simulink model "untitled2"  (Simulink 7.6)
settings: Solver=ode4  StartTime=0.0  StopTime=inf  FixedStep=0.2  RelTol=1e-3
undefined symbols (not defined in the file or in its folder): bit, Standard
libraries: xpclib x9, simulink x2
settings Model: xpc_rtwmakecfg_data=_xpccanac2pci_  Creator=Administrator  LastModifiedBy=Administrator  SimulationMode=external  BufferReuse=off
settings OptimizationCC: BlockReduction=off  OptimizeBlockIOStorage=off  BufferReuse=off  ExpressionFolding=off  LocalBlockOutputs=off
settings HardwareCC: ProdIntDivRoundTo=Zero  ProdEndianess=LittleEndian  ProdHWDeviceType=Generic->32-bit x86 compatible
settings RTWCC: SystemTargetFile=xpctarget.tlc  TemplateMakefile=xpc_default_tmf  Description=xPC Target  ProcessScript=xpctarget_make_rtw_hook  RTWCompilerOptimization=On
settings xpcTargetCC: TargetFcnLib=ansi_tfl_table_tmw.mat  TargetFunctionLibrary=XPC_BLAS  ERTCodeCoverageTool=None  ParMdlRefBuildCompliant=on  CombineSignalStateStructs=off  PortableWordSizes=off  xPCLoadParamSetFile=off  xPCConcurrentTasks=off  xPCEnableSFAnimation=off

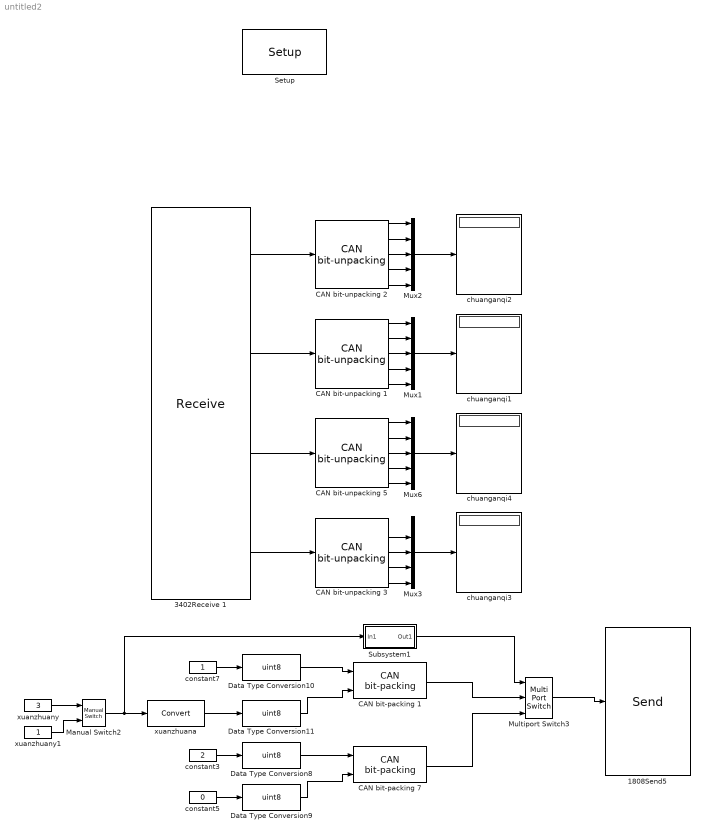
== system untitled2 ==
  1808Send5 : xpclib/CAN/Softing/CAN-AC2-PCI SJA 1000/Send   board=1  canPort=CAN 2  range=Standard (11-bit)  ids=1  sizes=[8]  output=off  ts=-1  ididx=[0]
  3402Receive 1 : xpclib/CAN/Softing/CAN-AC2-PCI SJA 1000/Receive   board=1  canPort=CAN 2  range=Standard (11-bit)  ids=[1 2 3 4]  lengths=8  output=Data  inten=off  ts=-1  ididx=[0,1,2,3]
  CAN bit-packing 1 : xpclib/CAN/Utilities/CAN bit-packing   bitpatterns={ [0:7] [8:15] }
  CAN bit-packing 7 : xpclib/CAN/Utilities/CAN bit-packing   bitpatterns={ [0:7] [8:15] }
  CAN bit-unpacking {1..3,5} (4 alike) : xpclib/CAN/Utilities/CAN bit-unpacking   bitpatterns={ [0:7],[8:15],[16:23],[24:31],[32:39]}  dtypes={ 'uint8','uint8','uint8','uint8','uint8' }
  Data Type Conversion{8..11} (4 alike) : DataTypeConversion  OutDataTypeStr=uint8
  Manual Switch2 : simulink/Signal Routing/Manual Switch  SystemSampleTime=-1  sw=1  action=0  varsize=off
  Multiport Switch3 : MultiPortSwitch  DataPortOrder=Zero-based contiguous  Inputs=2  zeroidx=on
  Mux{1..3,6} (4 alike) : Mux  Inputs=5
  "Setup " : xpclib/CAN/Softing/CAN-AC2-PCI SJA 1000/Setup   board=1  can1bus=Highspeed (ISO 11898)  can1Baudrate=500 kBaud  can1UserBR=[1,1,4,3]  can2bus=Highspeed (ISO 11898)  can2Baudrate=500 kBaud  can2UserBR=[1,1,4,3]  init=[]  term=[]  bus_off_out=off  bus_off_rec=Off  ioBaseAddress=-1
  Subsystem1 : Subsystem
  chuanganqi{1..4} (4 alike) : Display
  constant3 : Constant  Value=2
  constant5 : Constant  Value=0
  constant7 : Constant
  xuanzhuana : DataTypeConversion
  xuanzhuany : Constant  Value=3
  xuanzhuany1 : Constant
  wires:
  constant7/1 -> Data Type Conversion10/1
  Data Type Conversion10/1 -> CAN bit-packing 1/1
  Data Type Conversion11/1 -> CAN bit-packing 1/2
  constant3/1 -> Data Type Conversion8/1
  Data Type Conversion8/1 -> CAN bit-packing 7/1
  Data Type Conversion9/1 -> CAN bit-packing 7/2
  constant5/1 -> Data Type Conversion9/1
  xuanzhuana/1 -> Data Type Conversion11/1
  Multiport Switch3/1 -> 1808Send5/1
  CAN bit-packing 1/1 -> Multiport Switch3/2
  Subsystem1/1(Out1) -> Multiport Switch3/1
  CAN bit-packing 7/1 -> Multiport Switch3/3
  Manual Switch2/1 -> xuanzhuana/1, Subsystem1/1(In1)
  xuanzhuany/1 -> Manual Switch2/1
  xuanzhuany1/1 -> Manual Switch2/2
  CAN bit-unpacking 5/5 -> Mux6/5
  3402Receive 1/3 -> CAN bit-unpacking 5/1
  CAN bit-unpacking 5/1 -> Mux6/1
  CAN bit-unpacking 5/2 -> Mux6/2
  CAN bit-unpacking 5/3 -> Mux6/3
  CAN bit-unpacking 5/4 -> Mux6/4
  Mux6/1 -> chuanganqi4/1
  CAN bit-unpacking 1/5 -> Mux1/5
  CAN bit-unpacking 1/1 -> Mux1/1
  CAN bit-unpacking 1/2 -> Mux1/2
  CAN bit-unpacking 1/3 -> Mux1/3
  CAN bit-unpacking 1/4 -> Mux1/4
  Mux1/1 -> chuanganqi1/1
  3402Receive 1/2 -> CAN bit-unpacking 1/1
  CAN bit-unpacking 2/5 -> Mux2/5
  CAN bit-unpacking 2/1 -> Mux2/1
  CAN bit-unpacking 2/2 -> Mux2/2
  CAN bit-unpacking 2/3 -> Mux2/3
  CAN bit-unpacking 2/4 -> Mux2/4
  Mux2/1 -> chuanganqi2/1
  3402Receive 1/1 -> CAN bit-unpacking 2/1
  CAN bit-unpacking 3/5 -> Mux3/5
  CAN bit-unpacking 3/2 -> Mux3/2
  CAN bit-unpacking 3/3 -> Mux3/3
  CAN bit-unpacking 3/4 -> Mux3/4
  Mux3/1 -> chuanganqi3/1
  3402Receive 1/4 -> CAN bit-unpacking 3/1

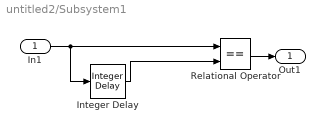
== system untitled2/Subsystem1 ==
  In1 : Inport
  Integer Delay : simulink/Discrete/Integer Delay  NumDelays=2  vinit=0.0  samptime=-1
  Relational Operator : RelationalOperator  Operator===  OutDataTypeStr=boolean
  Out1 : Outport
  wires:
  Integer Delay/1 -> Relational Operator/2
  In1/1 -> Integer Delay/1, Relational Operator/1
  Relational Operator/1 -> Out1/1
